simulink model "SizeDataCenterCoolingSystem"  (R2025b)
settings: Solver=daessc  StartTime=0.0  StopTime=31449600% hours ~ 8736  MaxStep=3600  RelTol=1e-3  AbsTol=1e-3
PreLoadFcn:
  | if ~exist("modelData")
  |     defaultGeographicalCoordinates;
  | end
undefined symbols (not defined in the file or in its folder): day, DiscIntNeverNeededParam, hour, modelData, month, value, year
libraries: fl_lib x63, nesl_utility x14, buildingEnergy_lib x13, datacenter_lib x5, simulink_extras x3, slpidlib x1
(part 2 of 2)

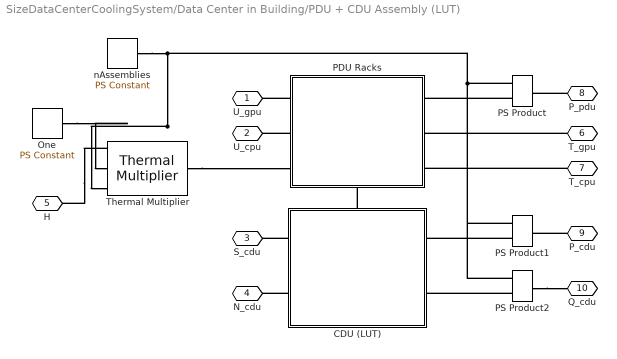
== system SizeDataCenterCoolingSystem/Data Center in Building/PDU + CDU Assembly (LUT) ==
  CDU (LUT) : Subsystem  mask{numPump=numPump, flowrate_vec=flowrate_vec, capacity_vec=capacity_vec, effPump_vec=effPump_vec, prDrop_mat=prDrop_mat, speed=speed}
      mask prompts: numPump "Total number of pumps (-)"; flowrate_vec "Coolant volumetric flowrate vector (m^3/s)"; capacity_vec "Heat exchanger capacity vector (W)"; effPump_vec "Pump efficiency vector, 0-1 (-)"; prDrop_mat "Pressure drop (Pa)"; speed "Pump speed scaling (-)"
      settings: CopyFcn=set_param(gcbh,'LinkStatus','none');  PortSchema="{\"entries\":[{\"content\":{\"sides\":[{\"content\":{\"connectorIds\":[\"LConn1\",\"LConn2\"]},\"type\":\"ConnectorPlacement.EquallySpacedRectSide\",\"uuid\":\"dd9276e8-a048-49df-a05c-f18b45aafce3\"},{\"content\":{\"connectorIds\":[\"RConn1\",\"RConn2\"],\"side\":\"RIGHT\"},\"type\":\"ConnectorPlacement.EquallySpacedRectSide\",\"uuid\":\"f4cbe01b-cfd4-4d60-aff7-a07955033ed5\"},{\"content\":{\"connectorIds\":[\"LConn3\"],\"side\":\"TOP\"},\"type\":\"ConnectorPlacement.EquallySpacedRectSide\",\"uuid\":\"ad27df56-4241-452c-8570-6a66062dd2f2\"}]},\"type\":\"ConnectorPlacement.EquallySpacedConnector\",\"uuid\":\"0333b5f9-1896-45e0-922d-790b0e5dd980\"}],\"packageUris\":[\"http://schema.mathworks.com/mf0/Connector/R2020b\"],\"version\":\"1.0\"}"
      mask Help: web("DocumentationCDULUT.html")
      mask DialogControl Container4 Prompt: CDU
      mask Display: image('icon_CDUtableBased.png');
  One : fl_lib/Physical Signals/Sources/PS Constant  constant=1
  PDU Racks : Subsystem  mask{nTrays=nTrays, nRacks=nRacks, trayMass=trayMass, trayCp=trayCp, trayThermalR=trayThermalR, nGPU=nGPU, gpuTDPperDie=gpuTDPperDie, gpuIdlePower=gpuIdlePower, gpuHBMpower=gpuHBMpower, gpuExponent=gpuExponent, gpuHBMutil=gpuHBMutil, gpuLeakage=gpuLeakage, gpuNominalDieT=gpuNominalDieT, gpuDieThermalC=gpuDieThermalC, gpuHeatSinkR=gpuHeatSinkR, gpuSurfArea=gpuSurfArea, gpuAmbientR=gpuAmbientR, nCPU=nCPU, cpuTDPperSocket=cpuTDPperSocket, cpuIdlePower=cpuIdlePower, cpuExponent=cpuExponent, cpuLeakage=cpuLeakage, cpuNominalDieT=cpuNominalDieT, cpuDieThermalC=cpuDieThermalC, cpuHeatSinkR=cpuHeatSinkR, cpuSurfArea=cpuSurfArea, cpuAmbientR=cpuAmbientR, initialT=initialT, htc=htc}
      mask prompts: nTrays "Number of IT trays per rack (-)"; nRacks "Number of racks (-)"; trayMass "Tray mass (kg)"; trayCp "Tray specific heat capacity (J/kg*K)"; trayThermalR "Tray to external thermal resistance (K/W)"; nGPU "Number of GPU per tray (-)"; gpuTDPperDie "GPU TDP per die (W)"; gpuIdlePower "GPU idle power (W)"; gpuHBMpower "HBM power per GPU (W)"; gpuExponent "GPU power utilization exponent (-)"; gpuHBMutil "HBM utilization as fraction of compute utilization (-)"; gpuLeakage "Leakage increase per K above nominal temperature (W/K)"; gpuNominalDieT "Nominal die temperature at TDP (K)"; gpuDieThermalC "GPU die thermal capacitance (J/K)"; gpuHeatSinkR "GPU die-heat-sink thermal resistance (K/W)"; gpuSurfArea "Surface area per die for ambient heat transfer (m^2)"; gpuAmbientR "GPU die-ambient thermal resistance (K/W)"; nCPU "Number of CPU per tray (-)"; cpuTDPperSocket "CPU TDP per socket (W)"; cpuIdlePower "CPU idle power per socket (W)"; cpuExponent "CPU power utilization exponent (-)"; cpuLeakage "Leakage increase per K above nominal temperature (W/K)"; cpuNominalDieT "Nominal die temperature at TDP (K)"; cpuDieThermalC "CPU die thermal capacitance (J/K)"; cpuHeatSinkR "CPU die-heat-sink thermal resistance (K/W)"; cpuSurfArea "Surface area per die for ambient heat transfer (m^2)"; cpuAmbientR "CPU die-ambient thermal resistance (K/W)"; initialT "Initial temperature (K)"; htc "Heat transfer coefficient to ambient (W/m^2.K)"
      settings: CopyFcn=set_param(gcbh,'LinkStatus','none');  PortSchema="{\"entries\":[{\"content\":{\"sides\":[{\"content\":{\"connectorIds\":[\"LConn1\",\"LConn2\",\"LConn3\"]},\"type\":\"ConnectorPlacement.EquallySpacedRectSide\",\"uuid\":\"1a9a884a-dab1-4495-bf62-c6b2de6c1039\"},{\"content\":{\"connectorIds\":[\"RConn1\",\"RConn2\",\"RConn3\"],\"side\":\"RIGHT\"},\"type\":\"ConnectorPlacement.EquallySpacedRectSide\",\"uuid\":\"05c53434-51c1-4fee-b885-c321dcda8b6b\"},{\"content\":{\"side\":\"TOP\"},\"type\":\"ConnectorPlacement.EquallySpacedRectSide\",\"uuid\":\"c7b5c534-d596-4858-a133-27f005e6c9d4\"},{\"content\":{\"connectorIds\":[\"RConn4\"],\"side\":\"BOTTOM\"},\"type\":\"ConnectorPlacement.EquallySpacedRectSide\",\"uuid\":\"693f3c99-4296-4d86-bfcc-da753d3e576f\"}]},\"type\":\"ConnectorPlacement.EquallySpacedConnector\",\"uuid\":\"ed91c467-c4d0-403f-af16-bac0257594fd\"}],\"packageUris\":[\"http://schema.mathworks.com/mf0/Connector/R2020b\"],\"version\":\"1.0\"}"
      mask Help: web("DocumentationPDURacks.html")
      mask DialogControl Container10 Prompt: PDU Racks
      mask DialogControl getRatingButton Prompt: Get Rating
      mask DialogControl Container9 Prompt: IT Tray
      mask DialogControl Container6 Prompt: GPU
      mask DialogControl Container7 Prompt: CPU
      mask DialogControl Container8 Prompt: Initial Conditions
      mask Display: image('icon_PDURacks.png');
  PS Product : fl_lib/Physical Signals/Functions/PS Product
  PS Product1 : fl_lib/Physical Signals/Functions/PS Product
  PS Product2 : fl_lib/Physical Signals/Functions/PS Product
  Thermal Multiplier : datacenter_lib/Thermal Multiplier
      settings: InternalSimscapePortConfiguration="{\"Bottom\":[],\"Left\":[{\"id\":\"A\",\"label\":\"A\",\"type\":\"foundation.thermal.thermal\"}],\"Right\":[{\"id\":\"B\",\"label\":\"B\",\"type\":\"foundation.thermal.thermal\"}],\"Top\":[{\"id\":\"Na\",\"label\":\"Na\",\"type\":\"input\"},{\"id\":\"Nb\",\"label\":\"Nb\",\"type\":\"input\"}]}"
  nAssemblies : fl_lib/Physical Signals/Sources/PS Constant  constant=nAssembly
  U_gpu : PMIOPort  Side=Left
  U_cpu : PMIOPort  Port=2  Side=Left
  S_cdu : PMIOPort  Port=3  Side=Left
  N_cdu : PMIOPort  Port=4  Side=Left
  H : PMIOPort  Port=5  Side=Left
  T_gpu : PMIOPort  Port=6  Side=Right
  T_cpu : PMIOPort  Port=7  Side=Right
  P_pdu : PMIOPort  Port=8  Side=Right
  P_cdu : PMIOPort  Port=9  Side=Right
  Q_cdu : PMIOPort  Port=10  Side=Right
  connections:
  P_cdu/RConn1 -- PS Product1/RConn1
  P_pdu/RConn1 -- PS Product/RConn1
  T_cpu/RConn1 -- PDU Racks/RConn3
  T_gpu/RConn1 -- PDU Racks/RConn2
  PS Product2/LConn2 -- CDU (LUT)/RConn2
  PS Product2/RConn1 -- Q_cdu/RConn1
  PS Product1/LConn2 -- CDU (LUT)/RConn1
  PS Product/LConn2 -- PDU Racks/RConn1
  One/RConn1 -- Thermal Multiplier/LConn2
  Thermal Multiplier/LConn3 -- PS Product/LConn1 -- PS Product1/LConn1 -- PS Product2/LConn1 -- nAssemblies/RConn1
  Thermal Multiplier/RConn1 -- PDU Racks/LConn3
  Thermal Multiplier/LConn1 -- H/RConn1
  PDU Racks/LConn2 -- U_cpu/RConn1
  CDU (LUT)/LConn1 -- S_cdu/RConn1
  PDU Racks/LConn1 -- U_gpu/RConn1
  CDU (LUT)/LConn3 -- PDU Racks/RConn4
  CDU (LUT)/LConn2 -- N_cdu/RConn1

== system SizeDataCenterCoolingSystem/Data Center in Building/Subsystem ==
  PS Max : fl_lib/Physical Signals/Nonlinear Operators/PS Max  ZeroCross=true
      settings: InternalSimscapePortConfiguration="{\"Bottom\":[],\"Left\":[{\"id\":\"I1\",\"label\":\"\",\"type\":\"input\"},{\"id\":\"I2\",\"label\":\"\",\"type\":\"input\"}],\"Right\":[{\"id\":\"O\",\"label\":\"\",\"type\":\"output\"}],\"Top\":[]}"
  "  " : PMIOPort  Side=Left
  "   " : PMIOPort  Port=2  Side=Left
  " " : PMIOPort  Port=3  Side=Right
  connections:
  PS Max/LConn2 -- "   "/RConn1
  PS Max/RConn1 -- " "/RConn1
  PS Max/LConn1 -- "  "/RConn1

== system SizeDataCenterCoolingSystem/Sensor/Subsystem1 ==
  S : Inport
  Discrete-Time Integrator : DiscreteIntegrator  gainval=1  InitialCondition=1  SampleTime=sampleTimeSec  ICPrevOutput=DiscIntNeverNeededParam  ICPrevScaledInput=DiscIntNeverNeededParam
  Divide : Product  Inputs=*/
  Subsystem : Subsystem
  R : Outport
  wires:
  Discrete-Time Integrator/1 -> Divide/1
  Subsystem/1(" ") -> Divide/2
  S/1 -> Discrete-Time Integrator/1
  Divide/1 -> R/1

== system SizeDataCenterCoolingSystem/Sensor/Subsystem2 ==
  S : Inport
  Discrete-Time Integrator : DiscreteIntegrator  gainval=1  InitialCondition=1  SampleTime=sampleTimeSec  ICPrevOutput=DiscIntNeverNeededParam  ICPrevScaledInput=DiscIntNeverNeededParam
  Divide : Product  Inputs=*/
  Subsystem : Subsystem
  R : Outport
  wires:
  Discrete-Time Integrator/1 -> Divide/1
  Subsystem/1(" ") -> Divide/2
  S/1 -> Discrete-Time Integrator/1
  Divide/1 -> R/1

== system SizeDataCenterCoolingSystem/Sensor/Subsystem3 ==
  S : Inport
  Discrete-Time Integrator : DiscreteIntegrator  gainval=1  InitialCondition=1  SampleTime=sampleTimeSec  ICPrevOutput=DiscIntNeverNeededParam  ICPrevScaledInput=DiscIntNeverNeededParam
  Divide : Product  Inputs=*/
  Subsystem : Subsystem
  R : Outport
  wires:
  Discrete-Time Integrator/1 -> Divide/1
  Subsystem/1(" ") -> Divide/2
  S/1 -> Discrete-Time Integrator/1
  Divide/1 -> R/1

== system SizeDataCenterCoolingSystem/Sensor/Subsystem4 ==
  S : Inport
  Discrete-Time Integrator : DiscreteIntegrator  gainval=1  InitialCondition=1  SampleTime=sampleTimeSec  ICPrevOutput=DiscIntNeverNeededParam  ICPrevScaledInput=DiscIntNeverNeededParam
  Divide : Product  Inputs=*/
  Subsystem : Subsystem
  R : Outport
  wires:
  Discrete-Time Integrator/1 -> Divide/1
  Subsystem/1(" ") -> Divide/2
  S/1 -> Discrete-Time Integrator/1
  Divide/1 -> R/1

== system SizeDataCenterCoolingSystem/Sensor/Subsystem5 ==
  S : Inport
  Discrete-Time Integrator : DiscreteIntegrator  gainval=1  InitialCondition=1  SampleTime=sampleTimeSec  ICPrevOutput=DiscIntNeverNeededParam  ICPrevScaledInput=DiscIntNeverNeededParam
  Divide : Product  Inputs=*/
  Subsystem : Subsystem
  R : Outport
  wires:
  Discrete-Time Integrator/1 -> Divide/1
  Subsystem/1(" ") -> Divide/2
  S/1 -> Discrete-Time Integrator/1
  Divide/1 -> R/1

== system SizeDataCenterCoolingSystem/Sensor/Subsystem6 ==
  S : Inport
  Discrete-Time Integrator : DiscreteIntegrator  gainval=1  InitialCondition=1  SampleTime=sampleTimeSec  ICPrevOutput=DiscIntNeverNeededParam  ICPrevScaledInput=DiscIntNeverNeededParam
  Divide : Product  Inputs=*/
  Subsystem : Subsystem
  R : Outport
  wires:
  Discrete-Time Integrator/1 -> Divide/1
  Subsystem/1(" ") -> Divide/2
  S/1 -> Discrete-Time Integrator/1
  Divide/1 -> R/1

== system SizeDataCenterCoolingSystem/Sensor/Subsystem7 ==
  S : Inport
  Discrete-Time Integrator : DiscreteIntegrator  gainval=1  InitialCondition=1  SampleTime=sampleTimeSec  ICPrevOutput=DiscIntNeverNeededParam  ICPrevScaledInput=DiscIntNeverNeededParam
  Divide : Product  Inputs=*/
  Subsystem : Subsystem
  R : Outport
  wires:
  Discrete-Time Integrator/1 -> Divide/1
  Subsystem/1(" ") -> Divide/2
  S/1 -> Discrete-Time Integrator/1
  Divide/1 -> R/1

== system SizeDataCenterCoolingSystem/Sensor/Subsystem9 ==
  S : Inport
  Discrete-Time Integrator : DiscreteIntegrator  gainval=1  InitialCondition=1  SampleTime=sampleTimeSec  ICPrevOutput=DiscIntNeverNeededParam  ICPrevScaledInput=DiscIntNeverNeededParam
  Divide : Product  Inputs=*/
  Subsystem : Subsystem
  R : Outport
  wires:
  Discrete-Time Integrator/1 -> Divide/1
  Subsystem/1(" ") -> Divide/2
  S/1 -> Discrete-Time Integrator/1
  Divide/1 -> R/1

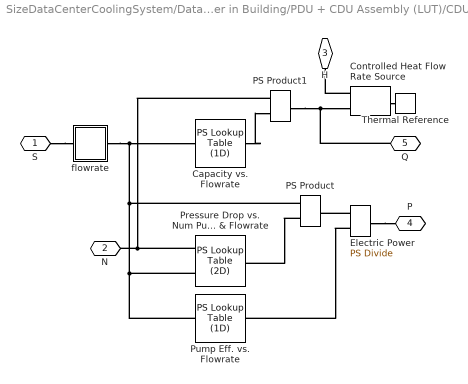
== system SizeDataCenterCoolingSystem/Data Center in Building/PDU + CDU Assembly (LUT)/CDU (LUT) ==
  Capacity vs. Flowrate : fl_lib/Physical Signals/Lookup Tables/PS Lookup Table (1D)  x=flowrate_vec m^3/s  f=capacity_vec W  interp_method=simscape.enum.interpolation.linear  extrap_method=simscape.enum.extrapolation.nearest
  Controlled Heat Flow Rate Source : fl_lib/Thermal/Thermal Sources/Controlled Heat Flow Rate Source
  Electric Power : fl_lib/Physical Signals/Functions/PS Divide
  PS Product : fl_lib/Physical Signals/Functions/PS Product
  PS Product1 : fl_lib/Physical Signals/Functions/PS Product
  Pressure Drop vs. Num Pump & Flowrate : fl_lib/Physical Signals/Lookup Tables/PS Lookup Table (2D)  x1=flowrate_vec m^3/s  x2=1:numPump  f=prDrop_mat Pa  interp_method=simscape.enum.interpolation.linear  extrap_method=simscape.enum.extrapolation.nearest
  Pump Eff. vs. Flowrate : fl_lib/Physical Signals/Lookup Tables/PS Lookup Table (1D)  x=flowrate_vec m^3/s  f=effPump_vec  interp_method=simscape.enum.interpolation.linear  extrap_method=simscape.enum.extrapolation.nearest
  Thermal Reference : fl_lib/Thermal/Thermal Elements/Thermal Reference
  flowrate : Subsystem
  S : PMIOPort  Side=Left
  N : PMIOPort  Port=2  Side=Left
  H : PMIOPort  Port=3  Side=Left
  P : PMIOPort  Port=4  Side=Right
  Q : PMIOPort  Port=5  Side=Right
  connections:
  Electric Power/LConn2 -- Pump Eff. vs. Flowrate/RConn1
  Controlled Heat Flow Rate Source/LConn1 -- Thermal Reference/LConn1
  PS Product1/LConn2 -- Pressure Drop vs. Num Pump & Flowrate/LConn2 -- N/RConn1
  PS Product/LConn1 -- Pressure Drop vs. Num Pump & Flowrate/RConn1
  Electric Power/RConn1 -- P/RConn1
  Electric Power/LConn1 -- PS Product/RConn1
  Controlled Heat Flow Rate Source/RConn2 -- H/RConn1
  Capacity vs. Flowrate/RConn1 -- PS Product1/LConn1
  PS Product1/RConn1 -- Q/RConn1 -- Controlled Heat Flow Rate Source/RConn1
  Pressure Drop vs. Num Pump & Flowrate/LConn1 -- Pump Eff. vs. Flowrate/LConn1 -- PS Product/LConn2 -- flowrate/RConn1 -- Capacity vs. Flowrate/LConn1
  S/RConn1 -- flowrate/LConn1

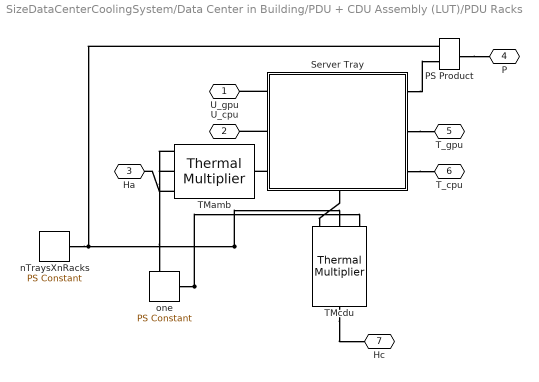
== system SizeDataCenterCoolingSystem/Data Center in Building/PDU + CDU Assembly (LUT)/PDU Racks ==
  PS Product : fl_lib/Physical Signals/Functions/PS Product
  Server Tray : Subsystem  mask{nGPU=nGPU, gpuTDPperDie=gpuTDPperDie, gpuIdlePower=gpuIdlePower, gpuHBMpower=gpuHBMpower, gpuExponent=gpuExponent, gpuHBMutil=gpuHBMutil, gpuLeakage=gpuLeakage, gpuNominalDieT=gpuLeakage, gpuDieThermalC=gpuDieThermalC, gpuHeatSinkR=gpuHeatSinkR, gpuSurfArea=gpuSurfArea, gpuAmbientR=gpuAmbientR, nCPU=nCPU, cpuTDPperSocket=cpuTDPperSocket, cpuIdlePower=cpuIdlePower, cpuExponent=cpuExponent, cpuLeakage=cpuLeakage, cpuNominalDieT=cpuNominalDieT, cpuDieThermalC=cpuDieThermalC, cpuHeatSinkR=cpuHeatSinkR, cpuSurfArea=cpuSurfArea, cpuAmbientR=cpuAmbientR, trayMass=trayMass, trayCp=trayCp, trayThermalR=trayThermalR, initialT=initialT, htc=htc}
      mask prompts: nGPU "Number of GPU (-)"; gpuTDPperDie "GPU TDP per die (W)"; gpuIdlePower "GPU idle power (W)"; gpuHBMpower "HBM power per GPU (W)"; gpuExponent "GPU power utilization exponent (-)"; gpuHBMutil "HBM utilization as fraction of compute utilization (-)"; gpuLeakage "Leakage increase per K above nominal temperature (W/K)"; gpuNominalDieT "Nominal die temperature at TDP (K)"; gpuDieThermalC "GPU die thermal capacitance (J/K)"; gpuHeatSinkR "GPU die-heat-sink thermal resistance (K/W)"; gpuSurfArea "Surface area per die for ambient heat transfer (m^2)"; gpuAmbientR "GPU die-ambient thermal resistance (K/W)"; nCPU "Number of CPU (-)"; cpuTDPperSocket "CPU TDP per socket (W)"; cpuIdlePower "CPU idle power per socket (W)"; cpuExponent "CPU power utilization exponent (-)"; cpuLeakage "Leakage increase per K above nominal temperature (W/K)"; cpuNominalDieT "Nominal die temperature at TDP (K)"; cpuDieThermalC "CPU die thermal capacitance (J/K)"; cpuHeatSinkR "CPU die-heat-sink thermal resistance (K/W)"; cpuSurfArea "Surface area per die for ambient heat transfer (m^2)"; cpuAmbientR "CPU die-ambient thermal resistance (K/W)"; trayMass "Tray mass (kg)"; trayCp "Tray specific heat capacity (J/kg*K)"; trayThermalR "Tray to external thermal resistance (K/W)"; initialT "Initial temperature (K)"; htc "Heat transfer coefficient to ambient (W/m^2.K)"
      settings: CopyFcn=set_param(gcbh,'LinkStatus','none');  PortSchema="{\"entries\":[{\"content\":{\"sides\":[{\"content\":{\"connectorIds\":[\"LConn1\",\"LConn2\",\"LConn3\"]},\"type\":\"ConnectorPlacement.EquallySpacedRectSide\",\"uuid\":\"893f21b9-92d6-433a-96e5-f8193a696c29\"},{\"content\":{\"connectorIds\":[\"RConn1\",\"RConn2\",\"RConn3\"],\"side\":\"RIGHT\"},\"type\":\"ConnectorPlacement.EquallySpacedRectSide\",\"uuid\":\"efd10409-70d8-4a6a-97a2-13f0e6f538e3\"},{\"content\":{\"side\":\"TOP\"},\"type\":\"ConnectorPlacement.EquallySpacedRectSide\",\"uuid\":\"8c9765cd-90e6-46de-916c-606bbb93143e\"},{\"content\":{\"connectorIds\":[\"RConn4\"],\"side\":\"BOTTOM\"},\"type\":\"ConnectorPlacement.EquallySpacedRectSide\",\"uuid\":\"9656b44e-d582-43b0-a7fe-c629821d6c27\"}]},\"type\":\"ConnectorPlacement.EquallySpacedConnector\",\"uuid\":\"add7a682-eb4b-4f46-a5b9-e161ccf96de5\"}],\"packageUris\":[\"http://schema.mathworks.com/mf0/Connector/R2020b\"],\"version\":\"1.0\"}"
      mask Help: web("DocumentationServerTray.html")
      mask DialogControl Container6 Prompt: GPU
      mask DialogControl Container7 Prompt: CPU
      mask DialogControl Container9 Prompt: IT Tray
      mask DialogControl Container8 Prompt: Initial Conditions
      mask Display: image('icon_serverPlate.png');
  TMamb : datacenter_lib/Thermal Multiplier
      settings: InternalSimscapePortConfiguration="{\"Bottom\":[],\"Left\":[{\"id\":\"A\",\"label\":\"A\",\"type\":\"foundation.thermal.thermal\"}],\"Right\":[{\"id\":\"B\",\"label\":\"B\",\"type\":\"foundation.thermal.thermal\"}],\"Top\":[{\"id\":\"Na\",\"label\":\"Na\",\"type\":\"input\"},{\"id\":\"Nb\",\"label\":\"Nb\",\"type\":\"input\"}]}"
  TMcdu : datacenter_lib/Thermal Multiplier
      settings: InternalSimscapePortConfiguration="{\"Bottom\":[],\"Left\":[{\"id\":\"A\",\"label\":\"A\",\"type\":\"foundation.thermal.thermal\"}],\"Right\":[{\"id\":\"B\",\"label\":\"B\",\"type\":\"foundation.thermal.thermal\"}],\"Top\":[{\"id\":\"Na\",\"label\":\"Na\",\"type\":\"input\"},{\"id\":\"Nb\",\"label\":\"Nb\",\"type\":\"input\"}]}"
  nTraysXnRacks : fl_lib/Physical Signals/Sources/PS Constant  constant=nTrays*nRacks
  one : fl_lib/Physical Signals/Sources/PS Constant  constant=1
  U_gpu : PMIOPort  Side=Left
  U_cpu : PMIOPort  Port=2  Side=Left
  Ha : PMIOPort  Port=3  Side=Left
  P : PMIOPort  Port=4  Side=Right
  T_gpu : PMIOPort  Port=5  Side=Right
  T_cpu : PMIOPort  Port=6  Side=Right
  Hc : PMIOPort  Port=7  Side=Right
  connections:
  Server Tray/LConn1 -- U_gpu/RConn1
  TMamb/LConn1 -- Ha/RConn1
  Server Tray/RConn2 -- T_gpu/RConn1
  TMcdu/RConn1 -- Hc/RConn1
  Server Tray/LConn2 -- U_cpu/RConn1
  Server Tray/RConn3 -- T_cpu/RConn1
  one/RConn1 -- TMcdu/LConn3 -- TMamb/LConn2
  Server Tray/RConn4 -- TMcdu/LConn1
  Server Tray/LConn3 -- TMamb/RConn1
  nTraysXnRacks/RConn1 -- PS Product/LConn1 -- TMcdu/LConn2 -- TMamb/LConn3
  Server Tray/RConn1 -- PS Product/LConn2
  PS Product/RConn1 -- P/RConn1

== system SizeDataCenterCoolingSystem/Sensor/Subsystem1/Subsystem ==
  Add : Sum
  Clock : Clock
  Constant : Constant  Value=1e-3
  " " : Outport
  wires:
  Constant/1 -> Add/1
  Clock/1 -> Add/2
  Add/1 -> " "/1

== system SizeDataCenterCoolingSystem/Sensor/Subsystem2/Subsystem ==
  Add : Sum
  Clock : Clock
  Constant : Constant  Value=1e-3
  " " : Outport
  wires:
  Constant/1 -> Add/1
  Clock/1 -> Add/2
  Add/1 -> " "/1

== system SizeDataCenterCoolingSystem/Sensor/Subsystem3/Subsystem ==
  Add : Sum
  Clock : Clock
  Constant : Constant  Value=1e-3
  " " : Outport
  wires:
  Constant/1 -> Add/1
  Clock/1 -> Add/2
  Add/1 -> " "/1

== system SizeDataCenterCoolingSystem/Sensor/Subsystem4/Subsystem ==
  Add : Sum
  Clock : Clock
  Constant : Constant  Value=1e-3
  " " : Outport
  wires:
  Constant/1 -> Add/1
  Clock/1 -> Add/2
  Add/1 -> " "/1

== system SizeDataCenterCoolingSystem/Sensor/Subsystem5/Subsystem ==
  Add : Sum
  Clock : Clock
  Constant : Constant  Value=1e-3
  " " : Outport
  wires:
  Constant/1 -> Add/1
  Clock/1 -> Add/2
  Add/1 -> " "/1

== system SizeDataCenterCoolingSystem/Sensor/Subsystem6/Subsystem ==
  Add : Sum
  Clock : Clock
  Constant : Constant  Value=1e-3
  " " : Outport
  wires:
  Constant/1 -> Add/1
  Clock/1 -> Add/2
  Add/1 -> " "/1

== system SizeDataCenterCoolingSystem/Sensor/Subsystem7/Subsystem ==
  Add : Sum
  Clock : Clock
  Constant : Constant  Value=1e-3
  " " : Outport
  wires:
  Constant/1 -> Add/1
  Clock/1 -> Add/2
  Add/1 -> " "/1

== system SizeDataCenterCoolingSystem/Sensor/Subsystem9/Subsystem ==
  Add : Sum
  Clock : Clock
  Constant : Constant  Value=1e-3
  " " : Outport
  wires:
  Constant/1 -> Add/1
  Clock/1 -> Add/2
  Add/1 -> " "/1

== system SizeDataCenterCoolingSystem/Data Center in Building/PDU + CDU Assembly (LUT)/CDU (LUT)/flowrate ==
  PS Product2 : fl_lib/Physical Signals/Functions/PS Product
  PS Saturation : fl_lib/Physical Signals/Nonlinear Operators/PS Saturation  upper_limit=speed  lower_limit=0  ZeroCross=true
  PS Subtract : fl_lib/Physical Signals/Functions/PS Subtract
  flowrate : fl_lib/Physical Signals/Functions/PS Add
  max_flowrate : fl_lib/Physical Signals/Sources/PS Constant  constant=max(flowrate_vec) m^3/s
  min_flowrate : fl_lib/Physical Signals/Sources/PS Constant  constant=min(flowrate_vec) m^3/s
  S : PMIOPort  Side=Left
  F : PMIOPort  Port=2  Side=Right
  connections:
  max_flowrate/RConn1 -- PS Subtract/LConn1
  PS Saturation/RConn1 -- PS Product2/LConn2
  PS Subtract/RConn1 -- PS Product2/LConn1
  flowrate/RConn1 -- F/RConn1
  min_flowrate/RConn1 -- PS Subtract/LConn2 -- flowrate/LConn2
  flowrate/LConn1 -- PS Product2/RConn1
  S/RConn1 -- PS Saturation/LConn1

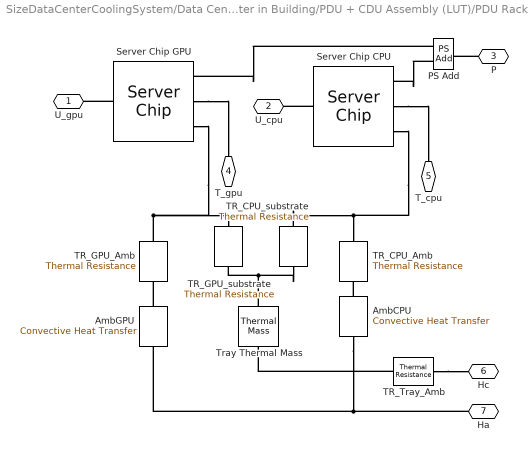
== system SizeDataCenterCoolingSystem/Data Center in Building/PDU + CDU Assembly (LUT)/PDU Racks/Server Tray ==
  AmbCPU : fl_lib/Thermal/Thermal Elements/Convective Heat Transfer  thermal_type=foundation.enum.constant_variable.constant  area=cpuSurfArea*nCPU m^2  heat_tr_coeff=htc W/(K*m^2)  min_heat_tr_coeff=1e-3 W/(K*m^2)  T_specify=off  T_priority=None  T=0 K  T_nominal_specify=off  T_nominal_value=1  T_nominal_unit=K  Q_specify=off  Q_priority=None  Q=0 W  Q_nominal_specify=off  Q_nominal_value=1  Q_nominal_unit=W
  AmbGPU : fl_lib/Thermal/Thermal Elements/Convective Heat Transfer  thermal_type=foundation.enum.constant_variable.constant  area=gpuSurfArea*nGPU m^2  heat_tr_coeff=htc W/(K*m^2)  min_heat_tr_coeff=1e-3 W/(K*m^2)  T_specify=off  T_priority=None  T=0 K  T_nominal_specify=off  T_nominal_value=1  T_nominal_unit=K  Q_specify=off  Q_priority=None  Q=0 W  Q_nominal_specify=off  Q_nominal_value=1  Q_nominal_unit=W
  PS Add : fl_lib/Physical Signals/Functions/PS Add
  Server Chip CPU : datacenter_lib/Server Chip  processorType=ProcessorType.CPU  numGPUs=4  numCPUs=nCPU  gpuTDP=1200 W  gpuIdlePower=300 W  gpuPowerExponent=1.4  hbmPowPerGPU=80 W  hbmUtilizationFrac=0.7  cpuTDP=cpuTDPperSocket W  cpuIdlePower=cpuIdlePower W  cpuPowerExponent=cpuExponent  PleakageCoeff=cpuLeakage W/K  chipTnominal=cpuNominalDieT K  chipCth=cpuDieThermalC J/K  T_specify=on  T_priority=High  T=initialT K  T_nominal_specify=off  T_nominal_value=1  T_nominal_unit=K  Q_specify=off  Q_priority=None  Q=0 W  Q_nominal_specify=off  Q_nominal_value=1  Q_nominal_unit=W
      settings: InternalSimscapePortConfiguration="{\"Bottom\":[{\"id\":\"H\",\"label\":\"H\",\"type\":\"foundation.thermal.thermal\"}],\"Left\":[{\"id\":\"U\",\"label\":\"U\",\"type\":\"input\"}],\"Right\":[{\"id\":\"Pow\",\"label\":\"P\",\"type\":\"output\"},{\"id\":\"Tchip\",\"label\":\"T\",\"type\":\"output\"}],\"Top\":[]}"
  Server Chip GPU : datacenter_lib/Server Chip  processorType=ProcessorType.GPU  numGPUs=nGPU  numCPUs=nCPU  gpuTDP=gpuTDPperDie W  gpuIdlePower=gpuIdlePower W  gpuPowerExponent=gpuExponent  hbmPowPerGPU=gpuHBMpower W  hbmUtilizationFrac=gpuHBMutil  cpuTDP=cpuTDPperSocket W  cpuIdlePower=cpuIdlePower W  cpuPowerExponent=1.1  PleakageCoeff=gpuLeakage W/K  chipTnominal=gpuNominalDieT K  chipCth=gpuDieThermalC J/K  T_specify=on  T_priority=High  T=initialT K  T_nominal_specify=off  T_nominal_value=1  T_nominal_unit=K  Q_specify=off  Q_priority=None  Q=0 W  Q_nominal_specify=off  Q_nominal_value=1  Q_nominal_unit=W
      settings: InternalSimscapePortConfiguration="{\"Bottom\":[{\"id\":\"H\",\"label\":\"H\",\"type\":\"foundation.thermal.thermal\"}],\"Left\":[{\"id\":\"U\",\"label\":\"U\",\"type\":\"input\"}],\"Right\":[{\"id\":\"Pow\",\"label\":\"P\",\"type\":\"output\"},{\"id\":\"Tchip\",\"label\":\"T\",\"type\":\"output\"}],\"Top\":[]}"
  TR_CPU_Amb : fl_lib/Thermal/Thermal Elements/Thermal Resistance  resistance=cpuAmbientR/nCPU K/W  T_specify=off  T_priority=None  T=0 K  T_nominal_specify=off  T_nominal_value=1  T_nominal_unit=K  Q_specify=off  Q_priority=None  Q=0 W  Q_nominal_specify=off  Q_nominal_value=1  Q_nominal_unit=W
  TR_CPU_substrate : fl_lib/Thermal/Thermal Elements/Thermal Resistance  resistance=cpuHeatSinkR/nCPU K/W  T_specify=off  T_priority=None  T=0 K  T_nominal_specify=off  T_nominal_value=1  T_nominal_unit=K  Q_specify=off  Q_priority=None  Q=0 W  Q_nominal_specify=off  Q_nominal_value=1  Q_nominal_unit=W
  TR_GPU_Amb : fl_lib/Thermal/Thermal Elements/Thermal Resistance  resistance=gpuAmbientR/nGPU K/W  T_specify=off  T_priority=None  T=0 K  T_nominal_specify=off  T_nominal_value=1  T_nominal_unit=K  Q_specify=off  Q_priority=None  Q=0 W  Q_nominal_specify=off  Q_nominal_value=1  Q_nominal_unit=W
  TR_GPU_substrate : fl_lib/Thermal/Thermal Elements/Thermal Resistance  resistance=gpuHeatSinkR/nGPU K/W  T_specify=off  T_priority=None  T=0 K  T_nominal_specify=off  T_nominal_value=1  T_nominal_unit=K  Q_specify=off  Q_priority=None  Q=0 W  Q_nominal_specify=off  Q_nominal_value=1  Q_nominal_unit=W
  TR_Tray_Amb : fl_lib/Thermal/Thermal Elements/Thermal Resistance  resistance=trayThermalR K/W  T_specify=off  T_priority=None  T=0 K  T_nominal_specify=off  T_nominal_value=1  T_nominal_unit=K  Q_specify=off  Q_priority=None  Q=0 W  Q_nominal_specify=off  Q_nominal_value=1  Q_nominal_unit=W
  Tray Thermal Mass : fl_lib/Thermal/Thermal Elements/Thermal Mass  mass_type=foundation.enum.constant_variable.constant  mass=trayMass kg  sp_heat=trayCp J/(K*kg)  mass_min=1e-6 kg  num_ports=foundation.enum.numPorts2.two  m_specify=off  m_priority=High  m=1 kg  m_nominal_specify=off  m_nominal_value=1  m_nominal_unit=kg  T_specify=on  T_priority=High  T=initialT K  T_nominal_specify=off  T_nominal_value=1  T_nominal_unit=K  Q_specify=off  Q_priority=None  Q=0 W  Q_nominal_specify=off  Q_nominal_value=1  Q_nominal_unit=W
      settings: InternalSimscapePortConfiguration="{\"Bottom\":[],\"Left\":[{\"id\":\"M\",\"label\":\"\",\"type\":\"foundation.thermal.thermal\"}],\"Right\":[{\"id\":\"N\",\"label\":\"\",\"type\":\"foundation.thermal.thermal\"}],\"Top\":[]}"
  U_gpu : PMIOPort  Side=Left
  U_cpu : PMIOPort  Port=2  Side=Left
  P : PMIOPort  Port=3  Side=Right
  T_gpu : PMIOPort  Port=4  Side=Right
  T_cpu : PMIOPort  Port=5  Side=Right
  Hc : PMIOPort  Port=6  Side=Right
  Ha : PMIOPort  Port=7  Side=Left
  connections:
  Tray Thermal Mass/LConn1 -- TR_GPU_substrate/RConn1 -- TR_CPU_substrate/RConn1
  Server Chip GPU/RConn2 -- T_gpu/RConn1
  TR_CPU_substrate/LConn1 -- TR_CPU_Amb/LConn1 -- Server Chip CPU/RConn3
  TR_GPU_Amb/RConn1 -- Server Chip GPU/RConn3 -- TR_GPU_substrate/LConn1
  TR_Tray_Amb/LConn1 -- Tray Thermal Mass/RConn1
  Server Chip GPU/LConn1 -- U_gpu/RConn1
  Server Chip CPU/LConn1 -- U_cpu/RConn1
  Server Chip CPU/RConn2 -- T_cpu/RConn1
  TR_Tray_Amb/RConn1 -- Hc/RConn1
  AmbGPU/LConn1 -- TR_GPU_Amb/LConn1
  AmbCPU/RConn1 -- AmbGPU/RConn1 -- Ha/RConn1
  P/RConn1 -- PS Add/RConn1
  PS Add/LConn1 -- Server Chip GPU/RConn1
  PS Add/LConn2 -- Server Chip CPU/RConn1
  AmbCPU/LConn1 -- TR_CPU_Amb/RConn1
